simulink model "lab1_1"  (R2016b)
settings: Solver=VariableStepAuto  StartTime=0.0  StopTime=10.0  MaxStep=0.01  MinStep=0.001  RelTol=1e-3
settings Model: Creator=Emanuel  LastModifiedBy=Emanuel
settings SolverCC: InitialStep=0.01

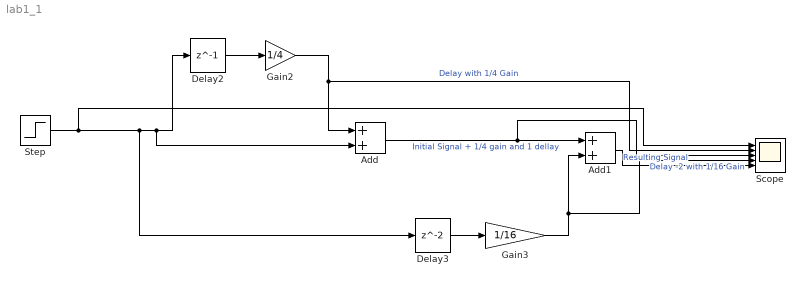
== system lab1_1 ==
  Add : Sum
  Add1 : Sum
  Delay2 : Delay  DelayLength=1  InitialCondition=0  SampleTime=1
  Delay3 : Delay  InitialCondition=0  SampleTime=1
  Gain2 : Gain  Gain=1/4
  Gain3 : Gain  Gain=1/16
  Scope : Scope  NumInputPorts=5
  Step : Step  SampleTime=0
  wires:
  Step/1 -> Scope/1, Delay3/1, Delay2/1, Add/2
  Delay2/1 -> Gain2/1
  Gain2/1 -> Scope/2, Add/1  "Delay with 1/4 Gain"
  Add/1 -> Scope/3, Add1/1  "Initial Signal + 1/4 gain and 1 dellay"
  Delay3/1 -> Gain3/1
  Gain3/1 -> Scope/4, Add1/2  "Delay -2 with 1/16 Gain"
  Add1/1 -> Scope/5  "Resulting Signal"
